simulink model "diode_clamped_3_lvl"  (R2023a)
settings: Solver=FixedStepAuto  StartTime=0.0  StopTime=0.1  FixedStep=1e-5  RelTol=1e-3
libraries: spsIGBTDiodeLib x12, spsDiodeLib x6, simulink x6, spsSeriesRLCBranchLib x5, spsGroundLib x2, spsDCVoltageSourceLib x1, spsThreePhaseVIMeasurementLib x1, spspowerguiLib x1
settings Model: Creator=suresh  LastModifiedBy=dhana

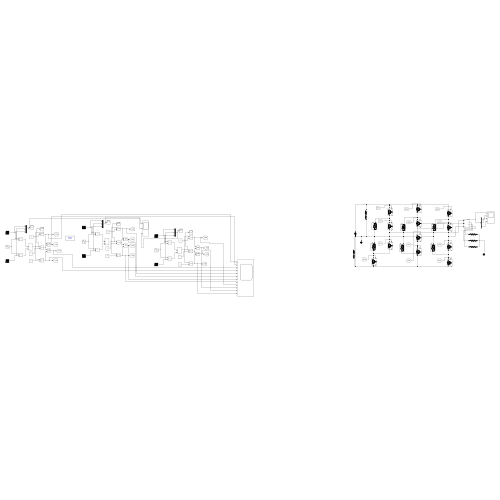
[thumbnail: Simulink's stored preview of the top-level diagram]
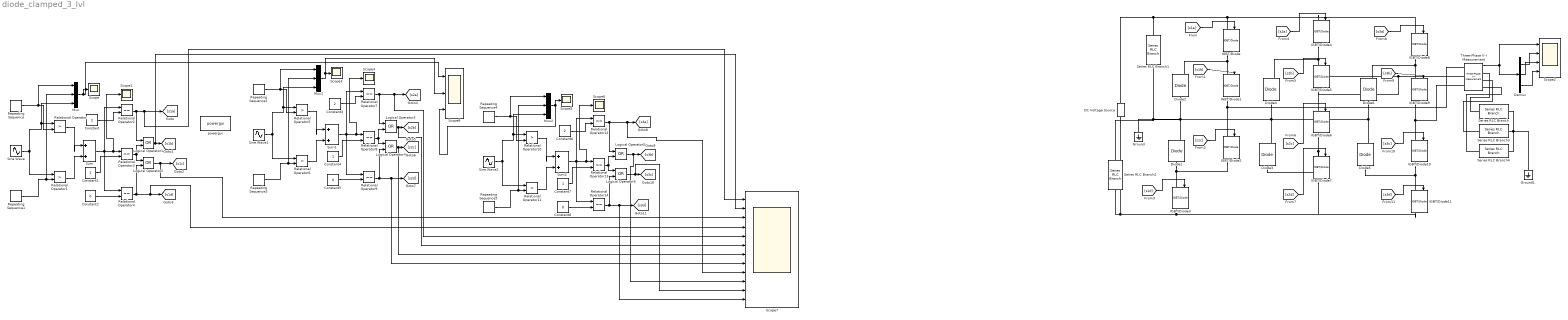
== system diode_clamped_3_lvl ==
  Constant : Constant  Value=2
  Constant1 : Constant
  Constant2 : Constant  Value=0
  Constant3 : Constant  Value=2
  Constant4 : Constant
  Constant5 : Constant  Value=0
  Constant6 : Constant  Value=2
  Constant7 : Constant
  Constant8 : Constant  Value=0
  DC Voltage Source : spsDCVoltageSourceLib/DC Voltage Source  Amplitude=100  Measurements=Voltage
  Demux : Demux  Outputs=3
  Diode{1..6} (6 alike) : spsDiodeLib/Diode  Ron=0.001  Lon=0  Vf=0.8  IC=0  UseSnubber=0  Rs=500  Cs=250e-9  Measurements=on
  Ground : spsGroundLib/Ground  LConnTagsString=a
  Ground1 : spsGroundLib/Ground  LConnTagsString=a
  IGBT/Diode{,1..11} (12 alike) : spsIGBTDiodeLib/IGBT//Diode  Ron=1e-3  Rs=1e5  Cs=inf  Measurements=on
  Logical Operator{1..6} (6 alike) : Logic  Operator=OR  AllPortsSameDT=off  OutDataTypeStr=boolean
  Mux : Mux  Inputs=3
  Mux1 : Mux  Inputs=3
  Mux2 : Mux  Inputs=3
  Relational Operator{,1,5..6,10..11} (6 alike) : RelationalOperator  Operator=>  OutDataTypeStr=boolean  RndMeth=Simplest  InputSameDT=off
  Relational Operator{2..4,7..9,12..14} (9 alike) : RelationalOperator  Operator===  OutDataTypeStr=boolean  RndMeth=Simplest  InputSameDT=off
  Repeating Sequence : simulink/Sources/Repeating Sequence  rep_seq_t=[0 1 2]*(1/1000)  rep_seq_y=[0 1 0]
  Repeating Sequence1 : simulink/Sources/Repeating Sequence  rep_seq_t=[0 1 2]*(1/1000)  rep_seq_y=[-1 0 -1]
  Repeating Sequence2 : simulink/Sources/Repeating Sequence  rep_seq_t=[0 1 2]*(1/1000)  rep_seq_y=[0 1 0]
  Repeating Sequence3 : simulink/Sources/Repeating Sequence  rep_seq_t=[0 1 2]*(1/1000)  rep_seq_y=[-1 0 -1]
  Repeating Sequence4 : simulink/Sources/Repeating Sequence  rep_seq_t=[0 1 2]*(1/1000)  rep_seq_y=[0 1 0]
  Repeating Sequence5 : simulink/Sources/Repeating Sequence  rep_seq_t=[0 1 2]*(1/1000)  rep_seq_y=[-1 0 -1]
  Scope{,1,3..6} (6 alike) : Scope
  Scope2 : Scope  NumInputPorts=4
  Scope7 : Scope  NumInputPorts=12
  Scope8 : Scope  NumInputPorts=3
  Series RLC Branch : spsSeriesRLCBranchLib/Series RLC Branch  LConnTagsString=__new0  RConnTagsString=__new0  BranchType=R  Resistance=500  Inductance=1e-3  SetiL0=off  InitialCurrent=0  Capacitance=1e-6  Setx0=off  InitialVoltage=0  Measurements=Branch voltage
  Series RLC Branch1 : spsSeriesRLCBranchLib/Series RLC Branch  LConnTagsString=__new0  RConnTagsString=__new0  BranchType=RC  Resistance=0.05  Inductance=1e-3  SetiL0=off  InitialCurrent=0  Capacitance=4.7e-3  Setx0=off  InitialVoltage=0  Measurements=Branch voltage and current
  Series RLC Branch2 : spsSeriesRLCBranchLib/Series RLC Branch  LConnTagsString=__new0  RConnTagsString=__new0  BranchType=RC  Resistance=0.05  Inductance=1e-3  SetiL0=off  InitialCurrent=0  Capacitance=4.7e-3  Setx0=off  InitialVoltage=0  Measurements=Branch voltage and current
  Series RLC Branch3 : spsSeriesRLCBranchLib/Series RLC Branch  LConnTagsString=__new0  RConnTagsString=__new0  BranchType=R  Resistance=100  Inductance=1e-3  SetiL0=off  InitialCurrent=0  Capacitance=1e-6  Setx0=off  InitialVoltage=0  Measurements=Branch voltage
  Series RLC Branch4 : spsSeriesRLCBranchLib/Series RLC Branch  LConnTagsString=__new0  RConnTagsString=__new0  BranchType=R  Resistance=250  Inductance=1e-3  SetiL0=off  InitialCurrent=0  Capacitance=1e-6  Setx0=off  InitialVoltage=0  Measurements=Branch voltage
  Sine Wave : Sin  Frequency=2*pi*50  SampleTime=0
  Sine Wave1 : Sin  Frequency=2*pi*50  Phase=4*pi/3  SampleTime=0
  Sine Wave2 : Sin  Frequency=2*pi*50  Phase=2*pi/3  SampleTime=0
  Sum : Sum  Inputs=|++
  Sum1 : Sum  Inputs=|++
  Sum2 : Sum  Inputs=|++
  Three-Phase V-I Measurement : spsThreePhaseVIMeasurementLib/Three-Phase V-I Measurement  VoltageMeasurement=phase-to-ground  SetLabelV=off  LabelV=Vabc  Vpu=off  VpuLL=off  CurrentMeasurement=no  SetLabelI=off  LabelI=Iabc  Ipu=off  Pbase=100e6  Vbase=500e3  OutputType=Complex  PhasorSimulation=off  PSBequivalent=0
  powergui : spspowerguiLib/powergui  Priority=1  SimulationMode=Discrete  SampleTime=1e-5  frequency=60  Iterations=50  frequencyindice=0  Pbase=100e6  ErrMax=1e-4  UnitsV=kV  UnitsW=MW  buscounter=0  FunctionMessages=off  echomessages=off  EnableUseOfTLC=off  CurrentSourceSwitches=off  DisableSnubberDevices=off  DisableRonSwitches=off  DisableVfSwitches=off  DisplayEquations=off  AutomaticDiscreteSolvers=off  SolverType=Tustin/Backward Euler (TBE)  Interpol=off  ExternalGateDelay=off  methode=off  Ts=100  x0status=blocks  SPID=on  SwTol=0  HookPort=off  NonlinearTolerance=1e-4  nMaxIteration=100  ContinueOnMaxIteration=off  RestoreLinks=warning  ResistiveCurrentMeasurement=off  Frange=[0:2:500]  Ylog=off  Xlog=on  ShowGrid=off  save=off  variable=ZData  structure=0  ZoomFFT=off  StartTime=0.0  cycles=1  DisplayStyle=1  fundamental=60  FreqAxis=off  MaxFrequency=1000  frequencyindicesteady=1  RmsSteady=1  display=off
  wires:
  Three-Phase V-I Measurement/1 -> Demux/1, Scope2/1
  Repeating Sequence/1 -> Relational Operator/2, Mux/1
  Sine Wave/1 -> Relational Operator1/1, Relational Operator/1, Mux/3
  Repeating Sequence1/1 -> Mux/2, Relational Operator1/2
  Relational Operator/1 -> Sum/1
  Relational Operator1/1 -> Sum/2
  Sum/1 -> Relational Operator4/1, Scope1/1, Relational Operator3/1, Relational Operator2/1
  Constant2/1 -> Relational Operator4/2
  Constant1/1 -> Relational Operator3/2
  Constant/1 -> Relational Operator2/2
  Relational Operator2/1 -> Scope7/1, [s1a], Logical Operator1/1
  Relational Operator4/1 -> Scope7/4, [s1d], Logical Operator2/2
  Relational Operator3/1 -> Logical Operator1/2, Logical Operator2/1
  Logical Operator2/1 -> Scope7/3, [s1c]
  Logical Operator1/1 -> Scope7/2, [s1b]
  [s1a] -> IGBT/Diode/1
  [s1b] -> IGBT/Diode1/1
  [s1c] -> IGBT/Diode2/1
  [s1d] -> IGBT/Diode3/1
  [s2d] -> IGBT/Diode7/1
  [s2c] -> IGBT/Diode6/1
  [s2b] -> IGBT/Diode5/1
  [s2a] -> IGBT/Diode4/1
  [s3a] -> IGBT/Diode8/1
  [s3b] -> IGBT/Diode9/1
  [s3c] -> IGBT/Diode10/1
  [s3d] -> IGBT/Diode11/1
  Mux1/1 -> Scope8/2, Scope3/1
  Logical Operator3/1 -> Scope7/6, [s2b]
  Logical Operator4/1 -> Scope7/7, [s2c]
  Relational Operator8/1 -> Logical Operator4/1, Logical Operator3/2
  Relational Operator9/1 -> Logical Operator4/2, Scope7/8, [s2d]
  Relational Operator7/1 -> Logical Operator3/1, Scope7/5, [s2a]
  Constant3/1 -> Relational Operator7/2
  Constant4/1 -> Relational Operator8/2
  Constant5/1 -> Relational Operator9/2
  Sum1/1 -> Relational Operator7/1, Relational Operator8/1, Scope4/1, Relational Operator9/1
  Relational Operator6/1 -> Sum1/2
  Relational Operator5/1 -> Sum1/1
  Repeating Sequence3/1 -> Relational Operator6/2, Mux1/2
  Sine Wave1/1 -> Mux1/3, Relational Operator5/1, Relational Operator6/1
  Repeating Sequence2/1 -> Mux1/1, Relational Operator5/2
  Demux/1 -> Scope2/2
  Demux/2 -> Scope2/3
  Demux/3 -> Scope2/4
  Logical Operator5/1 -> Scope7/10, [s3b]
  Mux2/1 -> Scope5/1, Scope8/3
  Constant7/1 -> Relational Operator13/2
  Relational Operator13/1 -> Logical Operator5/2, Logical Operator6/1
  Constant6/1 -> Relational Operator12/2
  Relational Operator12/1 -> Scope7/9, [s3a], Logical Operator5/1
  Relational Operator14/1 -> Scope7/12, [s3d], Logical Operator6/2
  Logical Operator6/1 -> Scope7/11, [s3c]
  Relational Operator10/1 -> Sum2/1
  Sum2/1 -> Relational Operator14/1, Scope6/1, Relational Operator13/1, Relational Operator12/1
  Constant8/1 -> Relational Operator14/2
  Relational Operator11/1 -> Sum2/2
  Repeating Sequence5/1 -> Mux2/2, Relational Operator11/2
  Repeating Sequence4/1 -> Relational Operator10/2, Mux2/1
  Sine Wave2/1 -> Relational Operator11/1, Relational Operator10/1, Mux2/3
  Mux/1 -> Scope8/1, Scope/1
  connections:
  Diode6/LConn1 -- Diode5/RConn1 -- Diode3/RConn1 -- Diode4/LConn1 -- Diode1/RConn1 -- Diode2/LConn1 -- Ground/LConn1 -- Series RLC Branch2/LConn1 -- Series RLC Branch1/RConn1
  DC Voltage Source/RConn1 -- IGBT/Diode4/LConn1 -- IGBT/Diode8/LConn1 -- IGBT/Diode/LConn1 -- Series RLC Branch1/LConn1
  DC Voltage Source/LConn1 -- IGBT/Diode11/RConn1 -- IGBT/Diode7/RConn1 -- IGBT/Diode3/RConn1 -- Series RLC Branch2/RConn1
  IGBT/Diode/RConn1 -- Diode2/RConn1 -- IGBT/Diode1/LConn1
  IGBT/Diode2/RConn1 -- Diode1/LConn1 -- IGBT/Diode3/LConn1
  IGBT/Diode1/RConn1 -- Three-Phase V-I Measurement/LConn1 -- IGBT/Diode2/LConn1
  Diode4/RConn1 -- IGBT/Diode5/LConn1 -- IGBT/Diode4/RConn1
  Diode3/LConn1 -- IGBT/Diode6/RConn1 -- IGBT/Diode7/LConn1
  IGBT/Diode5/RConn1 -- Three-Phase V-I Measurement/LConn2 -- IGBT/Diode6/LConn1
  IGBT/Diode8/RConn1 -- Diode6/RConn1 -- IGBT/Diode9/LConn1
  IGBT/Diode10/RConn1 -- Diode5/LConn1 -- IGBT/Diode11/LConn1
  IGBT/Diode9/RConn1 -- Three-Phase V-I Measurement/LConn3 -- IGBT/Diode10/LConn1
  Series RLC Branch/RConn1 -- Ground1/LConn1 -- Series RLC Branch4/RConn1 -- Series RLC Branch3/RConn1
  Series RLC Branch/LConn1 -- Three-Phase V-I Measurement/RConn1
  Series RLC Branch3/LConn1 -- Three-Phase V-I Measurement/RConn2
  Series RLC Branch4/LConn1 -- Three-Phase V-I Measurement/RConn3
